simulink model "simscape_pendulum"  (R2017a)
settings: Solver=VariableStepAuto  StartTime=0.0  StopTime=10.0  RelTol=1e-3  AbsTol=1e-3
libraries: fl_lib x16, nesl_utility x3, wrap_angle_lib x2, sdl_lib x2
settings Model: Creator=Grant  LastModifiedBy=Grant
settings DataIOCC: SaveFormat=Array
settings SimscapeCC: SimscapeLogType=all  SimscapeLogDataHistory=10000

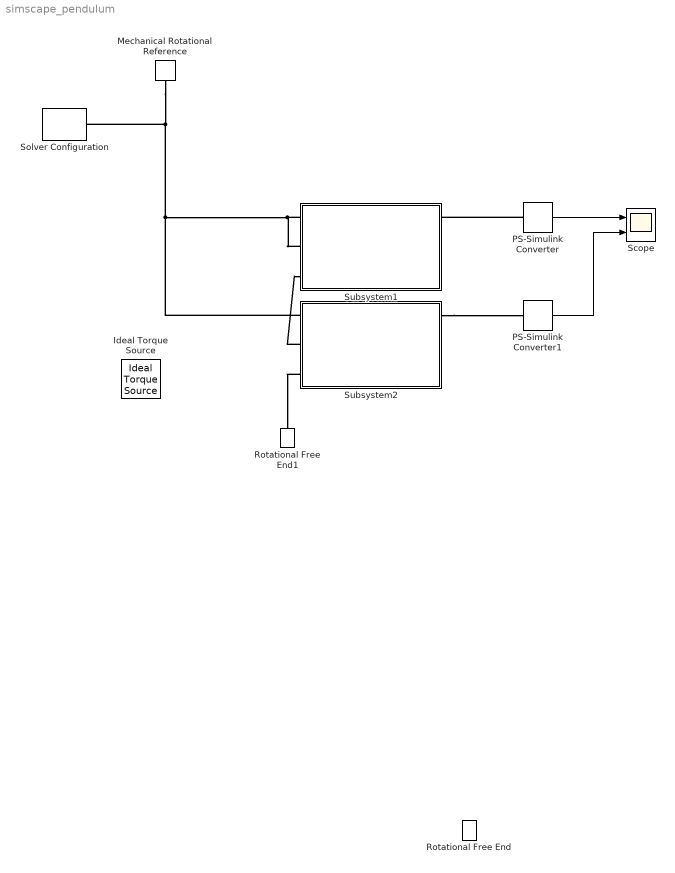
== system simscape_pendulum ==
  Ideal Torque Source : fl_lib/Mechanical/Mechanical Sources/Ideal Torque Source
  Mechanical Rotational Reference : fl_lib/Mechanical/Rotational Elements/Mechanical Rotational Reference
  PS-Simulink Converter : nesl_utility/PS-Simulink Converter  PhysicalDomain=network_engine_domain  SubClassName=ps_output  LeftPortType=input  RightPortType=output  PseudoPeriodic=off  Frequencies=[]  Unit=1  AffineConversion=off
  PS-Simulink Converter1 : nesl_utility/PS-Simulink Converter  PhysicalDomain=network_engine_domain  SubClassName=ps_output  LeftPortType=input  RightPortType=output  PseudoPeriodic=off  Frequencies=[]  Unit=1  AffineConversion=off
  Rotational Free End : fl_lib/Mechanical/Rotational Elements/Rotational Free End  w_specify=off  w_priority=None  w=0 rad/s  w_nominal_specify=off  w_nominal_unit=rad/s  w_nominal_value=1
      settings: SourceProductName=Simscape  SourceProductBaseCode=SS
  Rotational Free End1 : fl_lib/Mechanical/Rotational Elements/Rotational Free End  w_specify=off  w_priority=None  w=0 rad/s  w_nominal_specify=off  w_nominal_unit=rad/s  w_nominal_value=1
      settings: SourceProductName=Simscape  SourceProductBaseCode=SS
  Scope : Scope  NumInputPorts=2
  Solver Configuration : nesl_utility/Solver Configuration  PhysicalDomain=network_engine_domain  SubClassName=solver  LeftPortType=input  RightPortType=generic  Accelerate=off  Tones=[]  Harmonics=[]  SimulateNoise=off  Profile=off  UseLocalSampling=off  EnableSwitchedLinearOptims=on  FrequencyDomain=off  UseCCode=off  RelTol=0.001  AbsTol=1e-06  MinStep=1e-09  ToWorkspace=off  RevertToSquareIcSolve=off  NumHomotopyIterations=100  PhasorMode=off  PhasorModeNumHarmonics=1  OverrideAbsTol=off  DoDC=off  ResidualTolerance=1e-09  UseLocalSolver=off  LocalSolverChoice=NE_BACKWARD_EULER_ADVANCER  LocalSolverSampleTime=0.001  DoFixedCost=off  MaxNonlinIter=3  MaxModeIter=2  LinearAlgebra=Sparse  DelaysMemoryBudget=1024  AutomaticFiltering=on  FilteringTimeConstant=0.001
  Subsystem1 : Subsystem  mask{m=1, l=.01, b=.0001, g=-9.8, init_ang=pi/2}
      mask prompts: m "Mass"; l "Length"; b "Damping Ratio"; g "Gravity"; init_ang "Initial Angle"
  Subsystem2 : Subsystem  mask{m=1, l=.01, b=.0001, g=-9.8, init_ang=pi/2}
      mask prompts: m "Mass"; l "Length"; b "Damping Ratio"; g "Gravity"; init_ang "Initial Angle"
  wires:
  PS-Simulink Converter/1 -> Scope/1
  PS-Simulink Converter1/1 -> Scope/2
  connections:
  Mechanical Rotational Reference/LConn1 -- Subsystem2/LConn1 -- Subsystem1/LConn2 -- Subsystem1/LConn1 -- Solver Configuration/RConn1
  PS-Simulink Converter/LConn1 -- Subsystem1/RConn1
  Subsystem2/RConn1 -- PS-Simulink Converter1/LConn1
  Subsystem2/LConn2 -- Subsystem1/LConn3
  Subsystem2/LConn3 -- Rotational Free End1/LConn1

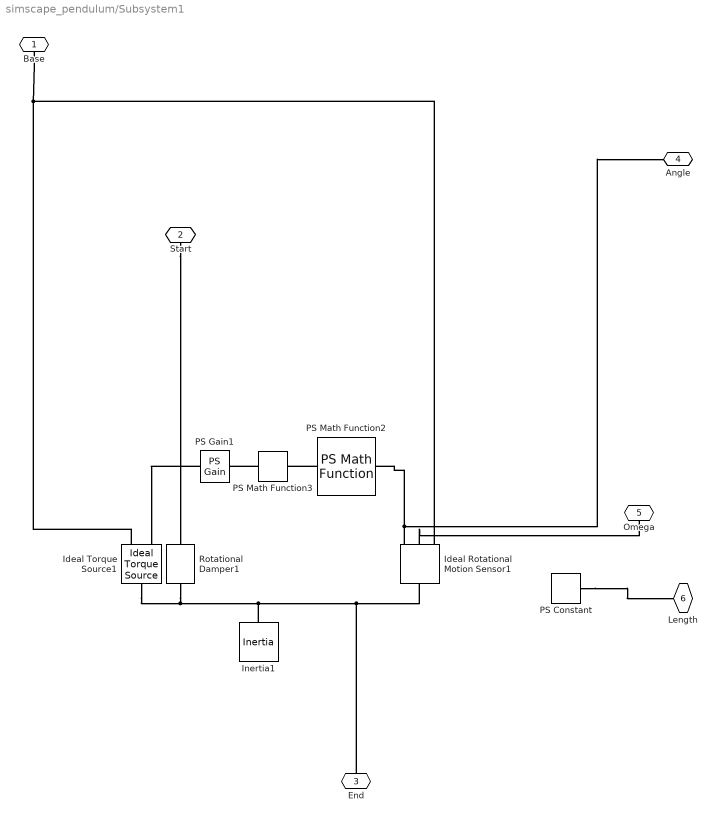
== system simscape_pendulum/Subsystem1 ==
  Ideal Rotational Motion Sensor1 : fl_lib/Mechanical/Mechanical Sensors/Ideal Rotational Motion Sensor  offset=init_ang rad
  Ideal Torque Source1 : fl_lib/Mechanical/Mechanical Sources/Ideal Torque Source
  Inertia1 : fl_lib/Mechanical/Rotational Elements/Inertia  inertia=m*l*l/3 kg*m^2  w_specify=off  w_priority=High  w=0 rad/s  w_nominal_specify=off  w_nominal_unit=rad/s  w_nominal_value=1  t_specify=off  t_priority=None  t=0 N*m  t_nominal_specify=off  t_nominal_unit=N*m  t_nominal_value=1
  PS Constant : fl_lib/Physical Signals/Sources/PS Constant  constant=l
  PS Gain1 : fl_lib/Physical Signals/Functions/PS Gain  gain=m*g*l/2
  PS Math Function2 : wrap_angle_lib/PS Math Function
  PS Math Function3 : fl_lib/Physical Signals/Functions/PS Math Function  fcn_choice=1
      settings: SourceProductName=Simscape  SourceProductBaseCode=SS
  Rotational Damper1 : sdl_lib/Couplings & Drives/Springs & Dampers/Rotational Damper  D=b N*m/(rad/s)  enable_faults=0  b_fault=100 N*m/(rad/s)  temporal_fault=0  fault_time=5 s  shock_fault=0  acceleration_limit=100 rad/s^2  shock_limit=1  report_fault=1
      settings: SourceProductName=Simscape Driveline  SourceProductBaseCode=LD
  Base : PMIOPort  Port=1  Side=Left
  Start : PMIOPort  Port=2  Side=Left
  End : PMIOPort  Port=3  Side=Left
  Angle : PMIOPort  Port=4  Side=Right
  Omega : PMIOPort  Port=5  Side=Right
  "Length " : PMIOPort  Port=6  Side=Right
  connections:
  Ideal Rotational Motion Sensor1/RConn2 -- Omega/RConn1
  Base/RConn1 -- Ideal Torque Source1/RConn2 -- Ideal Rotational Motion Sensor1/RConn1
  Start/RConn1 -- Rotational Damper1/RConn1
  PS Math Function3/RConn1 -- PS Gain1/LConn1
  Ideal Torque Source1/LConn1 -- Rotational Damper1/LConn1 -- Inertia1/LConn1 -- Ideal Rotational Motion Sensor1/LConn1 -- End/RConn1
  PS Gain1/RConn1 -- Ideal Torque Source1/RConn1
  PS Math Function2/RConn1 -- PS Math Function3/LConn1
  PS Math Function2/LConn1 -- Ideal Rotational Motion Sensor1/RConn3 -- Angle/RConn1
  PS Constant/RConn1 -- "Length "/RConn1

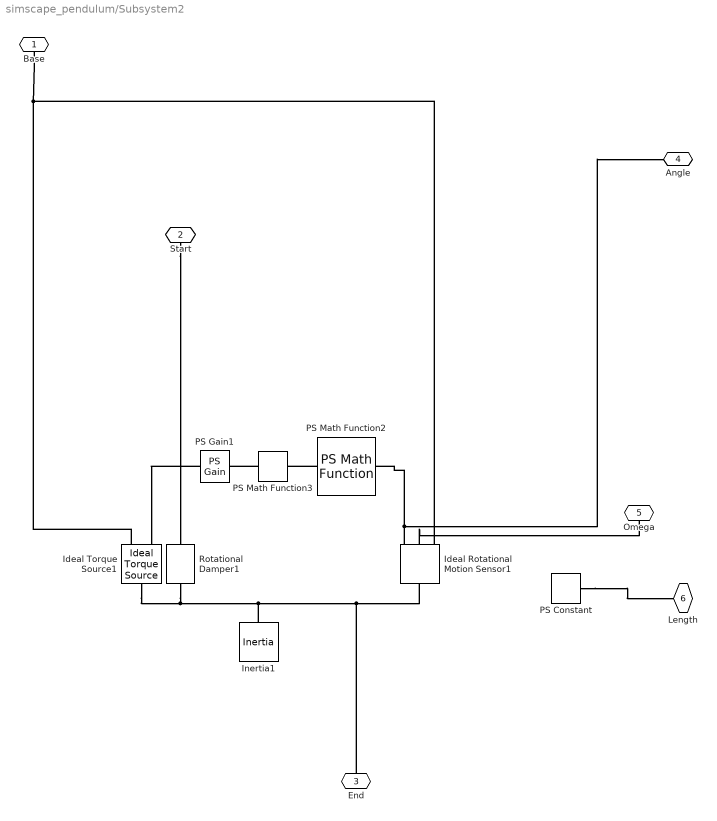
== system simscape_pendulum/Subsystem2 ==
  Ideal Rotational Motion Sensor1 : fl_lib/Mechanical/Mechanical Sensors/Ideal Rotational Motion Sensor  offset=init_ang rad
  Ideal Torque Source1 : fl_lib/Mechanical/Mechanical Sources/Ideal Torque Source
  Inertia1 : fl_lib/Mechanical/Rotational Elements/Inertia  inertia=m*l*l/3 kg*m^2  w_specify=off  w_priority=High  w=0 rad/s  w_nominal_specify=off  w_nominal_unit=rad/s  w_nominal_value=1  t_specify=off  t_priority=None  t=0 N*m  t_nominal_specify=off  t_nominal_unit=N*m  t_nominal_value=1
  PS Constant : fl_lib/Physical Signals/Sources/PS Constant  constant=l
  PS Gain1 : fl_lib/Physical Signals/Functions/PS Gain  gain=m*g*l/2
  PS Math Function2 : wrap_angle_lib/PS Math Function
  PS Math Function3 : fl_lib/Physical Signals/Functions/PS Math Function  fcn_choice=1
      settings: SourceProductName=Simscape  SourceProductBaseCode=SS
  Rotational Damper1 : sdl_lib/Couplings & Drives/Springs & Dampers/Rotational Damper  D=b N*m/(rad/s)  enable_faults=0  b_fault=100 N*m/(rad/s)  temporal_fault=0  fault_time=5 s  shock_fault=0  acceleration_limit=100 rad/s^2  shock_limit=1  report_fault=1
      settings: SourceProductName=Simscape Driveline  SourceProductBaseCode=LD
  Base : PMIOPort  Port=1  Side=Left
  Start : PMIOPort  Port=2  Side=Left
  End : PMIOPort  Port=3  Side=Left
  Angle : PMIOPort  Port=4  Side=Right
  Omega : PMIOPort  Port=5  Side=Right
  "Length " : PMIOPort  Port=6  Side=Right
  connections:
  Ideal Rotational Motion Sensor1/RConn2 -- Omega/RConn1
  Base/RConn1 -- Ideal Torque Source1/RConn2 -- Ideal Rotational Motion Sensor1/RConn1
  Start/RConn1 -- Rotational Damper1/RConn1
  PS Math Function3/RConn1 -- PS Gain1/LConn1
  Ideal Torque Source1/LConn1 -- Rotational Damper1/LConn1 -- Inertia1/LConn1 -- Ideal Rotational Motion Sensor1/LConn1 -- End/RConn1
  PS Gain1/RConn1 -- Ideal Torque Source1/RConn1
  PS Math Function2/RConn1 -- PS Math Function3/LConn1
  PS Math Function2/LConn1 -- Ideal Rotational Motion Sensor1/RConn3 -- Angle/RConn1
  PS Constant/RConn1 -- "Length "/RConn1
